simulink model "VCU_Modes"  (R2025b)
settings: Solver=FixedStepDiscrete  StartTime=0.0  StopTime=10.0  FixedStep=0.01  RelTol=1e-3
values from neighbouring files (symbols this model uses):
  c_VCU_BattCurrDrvThd = 100.0    [VCU_Modes.sldd]
  c_VCU_BattCurrDrvTime = 200.0    [VCU_Modes.sldd]
  c_VCU_BattCurrParkThd = 5.0    [VCU_Modes.sldd]
  c_VCU_BattCurrPeakDrvThd = 180.0    [VCU_Modes.sldd]
  c_VCU_BattSocDrvThd = 10.0    [VCU_Modes.sldd]
  c_VCU_BattSocLimpThd = 5.0    [VCU_Modes.sldd]
  c_VCU_BattTempDrvThdMax = 60.0    [VCU_Modes.sldd]
  c_VCU_BattTempParkThd = 45.0    [VCU_Modes.sldd]
  c_VCU_BattTempParkThdFlt = 55.0    [VCU_Modes.sldd]
  c_VCU_DrvThdWait = 100.0    [VCU_Modes.sldd]
  c_VCU_EcuTempDrvThdMax = 95.0    [VCU_Modes.sldd]
  c_VCU_EcuTempParkThd = 70.0    [VCU_Modes.sldd]
  c_VCU_EcuTempParkThdFlt = 85.0    [VCU_Modes.sldd]
  c_VCU_FailSafeThdTime = 200.0    [VCU_Modes.sldd]
  c_VCU_FrontLampExclusive_B = 0.0    [VCU_Modes.sldd]
  c_VCU_HeadLampAmbientThd = 300.0    [VCU_Modes.sldd]
  c_VCU_HeadlampAutoEnable_B = 1.0    [VCU_Modes.sldd]
  c_VCU_HeadlampManualOverride_B = 1.0    [VCU_Modes.sldd]
  c_VCU_LongPressTimeThd = 200.0    [VCU_Modes.sldd]
  c_VCU_MotTempDrvThdMax = 120.0    [VCU_Modes.sldd]
  c_VCU_MotTempParkThd = 80.0    [VCU_Modes.sldd]
  c_VCU_MotTempParkThdFlt = 100.0    [VCU_Modes.sldd]
  c_VCU_ParkExtThdWait = 100.0    [VCU_Modes.sldd]
  c_VCU_ParkThdWait = 100.0    [VCU_Modes.sldd]
  F32_ZERO = 0.0    [VCU_Modes.sldd]
  FALSE = 0.0    [VCU_Modes.sldd]
  TRUE = 1.0    [VCU_Modes.sldd]
  UI8_ZERO = 0.0    [VCU_Modes.sldd]
undefined symbols (not defined in the file or in its folder): POWER_MODE, SIG_STATUS, VCU_MODE
libraries: Sanu_Lib x9, simulink x1
(part 2 of 2)

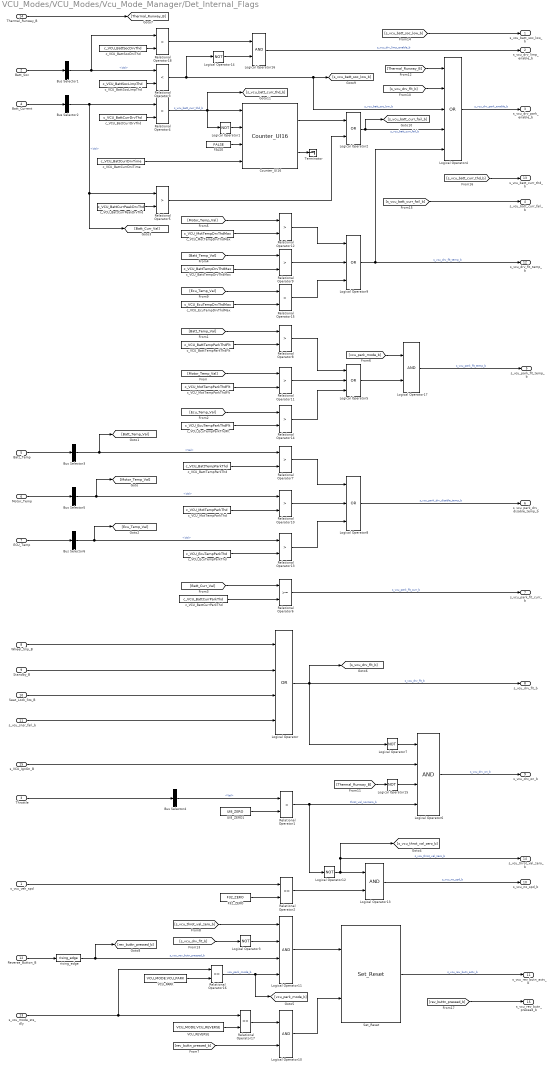
== system VCU_Modes/VCU_Modes/Vcu_Mode_Manager/Det_Internal_Flags ==
  s_vcu_veh_spd : Inport
  Batt_Soc : Inport  Port=2
  Throttle : Inport  Port=3
  Batt_Current : Inport  Port=4
  Batt_Temp : Inport  Port=5
  Motor_Temp : Inport  Port=6
  ECU_Temp : Inport  Port=7
  Wheel_Slip_B : Inport  Port=8
  Standby_B : Inport  Port=9
  Seat_Lock_Sts_B : Inport  Port=10
  s_vcu_snsr_fail_b : Inport  Port=11
  Reverse_Button_B : Inport  Port=12
  s_vcu_mode_sts_dly : Inport  Port=13
  Thermal_Runway_B : Inport  Port=14
  s_VCU_IgnOn_B : Inport  Port=15
  Bus Selector{1..6} (6 alike) : BusSelector  OutputSignals=Val
  Counter_UI16 : Sanu_Lib/Counter_UI16  SystemSampleTime=-1  VariantActivationTime=update diagram  EmptyChoice=off  PassThrough=off  PassThroughVariantControl=(default)  EmptyChoiceVariantControl=(default)  AllowFlexibleInterface=on  Latency=0  AutoFrameSizeCalculation=off
  F32_ZERO : Constant  Value=F32_ZERO  OutDataTypeStr=single  SampleTime=-1
  FALSE : Constant  Value=FALSE  OutDataTypeStr=boolean  SampleTime=-1
  Logical Operator : Logic  Operator=OR  Inputs=4  AllPortsSameDT=off  OutDataTypeStr=boolean
  Logical Operator{1,3,7,12,14..15} (6 alike) : Logic  Operator=NOT  AllPortsSameDT=off  OutDataTypeStr=boolean
  Logical Operator{10,13,16..17} (4 alike) : Logic  AllPortsSameDT=off  OutDataTypeStr=boolean
  Logical Operator11 : Logic  Inputs=4  AllPortsSameDT=off  OutDataTypeStr=boolean
  Logical Operator2 : Logic  Operator=OR  AllPortsSameDT=off  OutDataTypeStr=boolean
  Logical Operator4 : Logic  Operator=OR  Inputs=5  AllPortsSameDT=off  OutDataTypeStr=boolean
  Logical Operator5 : Logic  Operator=OR  Inputs=3  AllPortsSameDT=off  OutDataTypeStr=boolean
  Logical Operator6 : Logic  Inputs=4  AllPortsSameDT=off  OutDataTypeStr=boolean
  Logical Operator8 : Logic  Operator=OR  Inputs=3  AllPortsSameDT=off  OutDataTypeStr=boolean
  Logical Operator9 : Logic  Operator=OR  Inputs=3  AllPortsSameDT=off  OutDataTypeStr=boolean
  Relational Operator{1,4..5,7..15} (12 alike) : RelationalOperator  Operator=>  OutDataTypeStr=boolean  RndMeth=Simplest  InputSameDT=off
  Relational Operator16 : RelationalOperator  Operator===  OutDataTypeStr=boolean  RndMeth=Simplest  InputSameDT=off
  Relational Operator17 : RelationalOperator  Operator===  OutDataTypeStr=boolean  RndMeth=Simplest  InputSameDT=off
  Relational Operator18 : RelationalOperator  Operator=<  OutDataTypeStr=boolean  RndMeth=Simplest  InputSameDT=off
  Relational Operator2 : RelationalOperator  Operator===  OutDataTypeStr=boolean  RndMeth=Simplest  InputSameDT=off
  Relational Operator3 : RelationalOperator  Operator=<  OutDataTypeStr=boolean  RndMeth=Simplest  InputSameDT=off
  Relational Operator6 : RelationalOperator  OutDataTypeStr=boolean  RndMeth=Simplest  InputSameDT=off
  Set_Reset : Sanu_Lib/Set_Reset  SystemSampleTime=-1  VariantActivationTime=update diagram  EmptyChoice=off  PassThrough=off  PassThroughVariantControl=(default)  EmptyChoiceVariantControl=(default)  AllowFlexibleInterface=on  Latency=0  AutoFrameSizeCalculation=off
  Terminator : Terminator
  UI8_ZERO1 : Constant  Value=UI8_ZERO  OutDataTypeStr=uint8  SampleTime=-1
  VCU_PARK : Constant  Value=VCU_MODE.VCU_PARK  OutDataTypeStr=Enum: VCU_MODE  SampleTime=-1
  VCU_REVERSE : Constant  Value=VCU_MODE.VCU_REVERSE  OutDataTypeStr=Enum: VCU_MODE  SampleTime=-1
  c_VCU_BattCurrDrvThd : Constant  Value=c_VCU_BattCurrDrvThd  OutDataTypeStr=single  SampleTime=-1
  c_VCU_BattCurrDrvTime : Constant  Value=c_VCU_BattCurrDrvTime  OutDataTypeStr=uint16  SampleTime=-1
  c_VCU_BattCurrParkThd : Constant  Value=c_VCU_BattCurrParkThd  OutDataTypeStr=single  SampleTime=-1
  c_VCU_BattCurrPeakDrvThd : Constant  Value=c_VCU_BattCurrPeakDrvThd  OutDataTypeStr=single  SampleTime=-1
  c_VCU_BattSocDrvThd : Constant  Value=c_VCU_BattSocDrvThd  OutDataTypeStr=uint8  SampleTime=-1
  c_VCU_BattSocLimpThd : Constant  Value=c_VCU_BattSocLimpThd  OutDataTypeStr=uint8  SampleTime=-1
  c_VCU_BattTempDrvThdMax : Constant  Value=c_VCU_BattTempDrvThdMax  OutDataTypeStr=single  SampleTime=-1
  c_VCU_BattTempParkThd : Constant  Value=c_VCU_BattTempParkThd  OutDataTypeStr=single  SampleTime=-1
  c_VCU_BattTempParkThdFlt : Constant  Value=c_VCU_BattTempParkThdFlt  OutDataTypeStr=single  SampleTime=-1
  c_VCU_EcuTempDrvThdMax : Constant  Value=c_VCU_EcuTempDrvThdMax  OutDataTypeStr=single  SampleTime=-1
  c_VCU_EcuTempParkThd : Constant  Value=c_VCU_EcuTempParkThd  OutDataTypeStr=single  SampleTime=-1
  c_VCU_EcuTempParkThdFlt : Constant  Value=c_VCU_EcuTempParkThdFlt  OutDataTypeStr=single  SampleTime=-1
  c_VCU_MotTempDrvThdMax : Constant  Value=c_VCU_MotTempDrvThdMax  OutDataTypeStr=single  SampleTime=-1
  c_VCU_MotTempParkThd : Constant  Value=c_VCU_MotTempParkThd  OutDataTypeStr=single  SampleTime=-1
  c_VCU_MotTempParkThdFlt : Constant  Value=c_VCU_MotTempParkThdFlt  OutDataTypeStr=single  SampleTime=-1
  rising_edge : Sanu_Lib/rising_edge  SystemSampleTime=-1  VariantActivationTime=update diagram  EmptyChoice=off  PassThrough=off  PassThroughVariantControl=(default)  EmptyChoiceVariantControl=(default)  AllowFlexibleInterface=on  Latency=0  AutoFrameSizeCalculation=off
  s_vcu_batt_soc_low_b : Outport
  s_vcu_drv_limp_enable_b : Outport  Port=2
  s_vcu_drv_park_enable_b : Outport  Port=3
  s_vcu_batt_curr_fail_b : Outport  Port=4
  s_vcu_park_flt_temp_b : Outport  Port=5
  s_vcu_park_drv_disable_temp_b : Outport  Port=6
  s_vcu_park_flt_curr_b : Outport  Port=7
  s_vcu_drv_flt_b : Outport  Port=8
  s_vcu_drv_on_b : Outport  Port=9
  s_vcu_no_spd_b : Outport  Port=10
  s_vcu_rev_butn_actv_b : Outport  Port=11
  s_vcu_drv_flt_temp_b : Outport  Port=12
  s_vcu_batt_curr_thd_b : Outport  Port=13
  s_vcu_throt_val_zero_b : Outport  Port=14
  s_vcu_rev_butn_pressed_b : Outport  Port=15
  wires:
  [s_vcu_batt_soc_low_b] -> s_vcu_batt_soc_low_b/1
  Logical Operator16/1 -> s_vcu_drv_limp_enable_b/1  "s_vcu_drv_limp_enable_b"
  Relational Operator18/1 -> Logical Operator16/1
  Logical Operator14/1 -> Logical Operator16/2
  c_VCU_BattSocDrvThd/1 -> Relational Operator18/2
  [Thermal_Runway_B] -> Logical Operator4/1
  s_VCU_IgnOn_B/1 -> Logical Operator6/2
  Relational Operator6/1 -> s_vcu_park_flt_curr_b/1  "s_vcu_park_flt_curr_b"
  Logical Operator15/1 -> Logical Operator6/3
  [Thermal_Runway_B] -> Logical Operator15/1
  [rev_buttn_pressed_b] -> Logical Operator10/2
  [s_vcu_throt_val_zero_b] -> Logical Operator11/1
  Logical Operator3/1 -> Logical Operator11/2
  [s_vcu_drv_flt_b] -> Logical Operator3/1
  Logical Operator13/1 -> s_vcu_no_spd_b/1  "s_vcu_no_spd_b"
  [Ecu_Temp_Val] -> Relational Operator15/1
  Logical Operator4/1 -> s_vcu_drv_park_enable_b/1  "s_vcu_drv_park_enable_b"
  [Motor_Temp_Val] -> Relational Operator12/1
  Relational Operator9/1 -> Logical Operator9/2
  Logical Operator8/1 -> s_vcu_park_drv_disable_temp_b/1  "s_vcu_park_drv_disable_temp_b"
  Logical Operator/1 -> [s_vcu_drv_flt_b], s_vcu_drv_flt_b/1, Logical Operator7/1  "s_vcu_drv_flt_b"
  FALSE/1 -> Counter_UI16/3
  Relational Operator7/1 -> Logical Operator8/1
  Logical Operator1/1 -> Counter_UI16/2
  [Batt_Temp_Val] -> Relational Operator8/1
  Relational Operator16/1 -> [vcu_park_mode_b], Logical Operator11/4  "vcu_park_mode_b"
  Logical Operator11/1 -> Set_Reset/1
  Logical Operator7/1 -> Logical Operator6/1
  s_vcu_veh_spd/1 -> Relational Operator2/1
  c_VCU_EcuTempParkThdFlt/1 -> Relational Operator14/2
  Bus Selector6/1 -> Relational Operator13/1, [Ecu_Temp_Val]  "<Val>"
  s_vcu_snsr_fail_b/1 -> Logical Operator/4
  c_VCU_BattCurrPeakDrvThd/1 -> Relational Operator5/2
  c_VCU_BattTempParkThd/1 -> Relational Operator7/2
  ECU_Temp/1 -> Bus Selector6/1
  Seat_Lock_Sts_B/1 -> Logical Operator/3
  Logical Operator10/1 -> Set_Reset/2
  Relational Operator13/1 -> Logical Operator8/3
  c_VCU_BattCurrDrvTime/1 -> Counter_UI16/4
  Relational Operator11/1 -> Logical Operator5/2
  Relational Operator12/1 -> Logical Operator9/1
  [Batt_Temp_Val] -> Relational Operator9/1
  Logical Operator9/1 -> s_vcu_drv_flt_temp_b/1, Logical Operator4/5  "s_vcu_drv_flt_temp_b"
  c_VCU_BattCurrParkThd/1 -> Relational Operator6/2
  VCU_REVERSE/1 -> Relational Operator17/2
  Set_Reset/1 -> s_vcu_rev_butn_actv_b/1  "s_vcu_rev_butn_actv_b"
  VCU_PARK/1 -> Relational Operator16/2
  Counter_UI16/1 -> Logical Operator2/1
  [Ecu_Temp_Val] -> Relational Operator14/1
  Bus Selector1/1 -> Relational Operator3/1, Relational Operator18/1  "<Val>"
  Relational Operator2/1 -> Logical Operator13/2
  Relational Operator5/1 -> Logical Operator2/2
  Bus Selector5/1 -> Relational Operator10/1, [Motor_Temp_Val]  "<Val>"
  Batt_Soc/1 -> Bus Selector1/1
  [Motor_Temp_Val] -> Relational Operator11/1
  [s_vcu_drv_flt_b] -> Logical Operator4/2
  c_VCU_BattCurrDrvThd/1 -> Relational Operator4/2
  c_VCU_MotTempDrvThdMax/1 -> Relational Operator12/2
  Bus Selector3/1 -> Relational Operator7/1, [Batt_Temp_Val]  "<Val>"
  Relational Operator1/1 -> Logical Operator6/4, Logical Operator12/1  "throt_val_nonzero_b"
  c_VCU_MotTempParkThdFlt/1 -> Relational Operator11/2
  Batt_Temp/1 -> Bus Selector3/1
  Motor_Temp/1 -> Bus Selector5/1
  Relational Operator10/1 -> Logical Operator8/2
  rising_edge/1 -> Logical Operator11/3, [rev_buttn_pressed_b]  "s_vcu_rev_butn_pressed_b"
  c_VCU_MotTempParkThd/1 -> Relational Operator10/2
  Standby_B/1 -> Logical Operator/2
  Reverse_Button_B/1 -> rising_edge/1
  Wheel_Slip_B/1 -> Logical Operator/1
  Relational Operator17/1 -> Logical Operator10/1
  Throttle/1 -> Bus Selector4/1
  F32_ZERO/1 -> Relational Operator2/2
  [Batt_Curr_Val] -> Relational Operator6/1
  Relational Operator8/1 -> Logical Operator5/1
  c_VCU_BattSocLimpThd/1 -> Relational Operator3/2
  c_VCU_BattTempDrvThdMax/1 -> Relational Operator9/2
  Relational Operator15/1 -> Logical Operator9/3
  Logical Operator2/1 -> Logical Operator4/4, [s_vcu_batt_curr_fail_b]  "s_vcu_batt_curr_fail_b"
  Logical Operator6/1 -> s_vcu_drv_on_b/1  "s_vcu_drv_on_b"
  Counter_UI16/2 -> Terminator/1
  Bus Selector4/1 -> Relational Operator1/1  "<Val>"
  Logical Operator12/1 -> [s_vcu_throt_val_zero_b], s_vcu_throt_val_zero_b/1, Logical Operator13/1  "s_vcu_throt_val_zero_b"
  c_VCU_BattTempParkThdFlt/1 -> Relational Operator8/2
  c_VCU_EcuTempDrvThdMax/1 -> Relational Operator15/2
  Thermal_Runway_B/1 -> [Thermal_Runway_B]
  Relational Operator14/1 -> Logical Operator5/3
  Relational Operator4/1 -> [s_vcu_batt_curr_thd_b], Logical Operator1/1, Counter_UI16/1  "s_vcu_batt_curr_thd_b"
  Bus Selector2/1 -> Relational Operator4/1, Relational Operator5/1, [Batt_Curr_Val]  "<Val>"
  c_VCU_EcuTempParkThd/1 -> Relational Operator13/2
  UI8_ZERO1/1 -> Relational Operator1/2
  Batt_Current/1 -> Bus Selector2/1
  Relational Operator3/1 -> Logical Operator4/3, [s_vcu_batt_soc_low_b], Logical Operator14/1  "s_vcu_batt_soc_low_b"
  s_vcu_mode_sts_dly/1 -> Relational Operator16/1, Relational Operator17/1
  [vcu_park_mode_b] -> Logical Operator17/1
  [s_vcu_batt_curr_fail_b] -> s_vcu_batt_curr_fail_b/1
  [s_vcu_batt_curr_thd_b] -> s_vcu_batt_curr_thd_b/1
  Logical Operator5/1 -> Logical Operator17/2
  Logical Operator17/1 -> s_vcu_park_flt_temp_b/1  "s_vcu_park_flt_temp_b"
  [rev_buttn_pressed_b] -> s_vcu_rev_butn_pressed_b/1

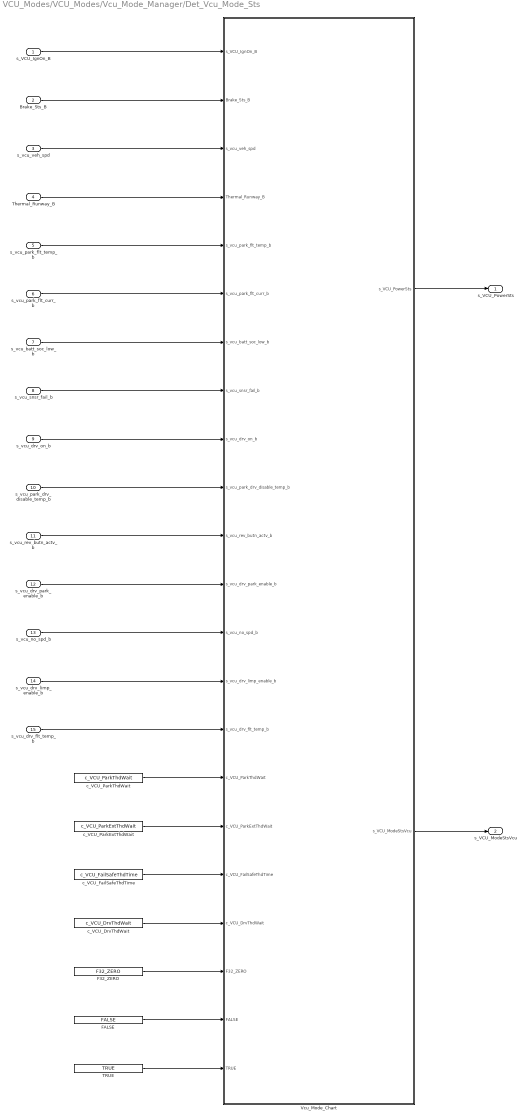
== system VCU_Modes/VCU_Modes/Vcu_Mode_Manager/Det_Vcu_Mode_Sts ==
  s_VCU_IgnOn_B : Inport
  Brake_Sts_B : Inport  Port=2
  s_vcu_veh_spd : Inport  Port=3
  Thermal_Runway_B : Inport  Port=4
  s_vcu_park_flt_temp_b : Inport  Port=5
  s_vcu_park_flt_curr_b : Inport  Port=6
  s_vcu_batt_soc_low_b : Inport  Port=7
  s_vcu_snsr_fail_b : Inport  Port=8
  s_vcu_drv_on_b : Inport  Port=9
  s_vcu_park_drv_disable_temp_b : Inport  Port=10
  s_vcu_rev_butn_actv_b : Inport  Port=11
  s_vcu_drv_park_enable_b : Inport  Port=12
  s_vcu_no_spd_b : Inport  Port=13
  s_vcu_drv_limp_enable_b : Inport  Port=14
  s_vcu_drv_flt_temp_b : Inport  Port=15
  F32_ZERO : Constant  Value=F32_ZERO  OutDataTypeStr=single  SampleTime=-1
  FALSE : Constant  Value=FALSE  OutDataTypeStr=boolean  SampleTime=-1
  TRUE : Constant  Value=TRUE  OutDataTypeStr=boolean  SampleTime=-1
  Vcu_Mode_Chart : Stateflow chart  TreatAsAtomicUnit=on
      settings: PortSchema="{\"entries\":[{\"content\":{\"sides\":[{\"content\":{\"connectorIds\":[\"In1\",\"In2\",\"In3\",\"In4\",\"In5\",\"In6\",\"In7\",\"In8\",\"In9\",\"In10\",\"In11\",\"In12\",\"In13\",\"In14\",\"In15\",\"In16\",\"In18\",\"In17\",\"In19\",\"In20\",\"In21\",\"In22\"]},\"type\":\"ConnectorPlacement.EquallySpacedRectSide\",\"uuid\":\"35025c92-f7ea-4c68-bbf7-eead624e483f\"},{\"content\":{\"connectorIds\":[\"Out1\",\"Out2\"],\"side\":\"RIGHT\"},\"type\":\"ConnectorPlacement.EquallySpacedRectSide\",\"uuid\":\"04b476af-775e-4130-9977-c38802426b78\"},{\"content\":{\"side\":\"TOP\"},\"type\":\"ConnectorPlacement.EquallySpacedRectSide\",\"uuid\":\"5327a217-51d4-4e1d-848e-3c1107d92c88\"}]},\"type\":\"ConnectorPlacement.EquallySpacedConnector\",\"uuid\":\"3867ef37-b688-49f3-9610-30f88bf37bff\"}],\"packageUris\":[\"http://schema.mathworks.com/mf0/Connector/R2020b\"],\"version\":\"1.0\"}"
  c_VCU_DrvThdWait : Constant  Value=c_VCU_DrvThdWait  OutDataTypeStr=uint16  SampleTime=-1
  c_VCU_FailSafeThdTime : Constant  Value=c_VCU_FailSafeThdTime  OutDataTypeStr=uint16  SampleTime=-1
  c_VCU_ParkExtThdWait : Constant  Value=c_VCU_ParkExtThdWait  OutDataTypeStr=uint16  SampleTime=-1
  c_VCU_ParkThdWait : Constant  Value=c_VCU_ParkThdWait  OutDataTypeStr=uint16  SampleTime=-1
  s_VCU_PowerSts : Outport
  s_VCU_ModeStsVcu : Outport  Port=2
  wires:
  s_VCU_IgnOn_B/1 -> Vcu_Mode_Chart/1(s_VCU_IgnOn_B)
  Brake_Sts_B/1 -> Vcu_Mode_Chart/2(Brake_Sts_B)
  Vcu_Mode_Chart/2(" s_VCU_ModeStsVcu") -> s_VCU_ModeStsVcu/1
  Vcu_Mode_Chart/1(s_VCU_PowerSts) -> s_VCU_PowerSts/1
  s_vcu_veh_spd/1 -> Vcu_Mode_Chart/3(s_vcu_veh_spd)
  Thermal_Runway_B/1 -> Vcu_Mode_Chart/4(Thermal_Runway_B)
  s_vcu_park_flt_temp_b/1 -> Vcu_Mode_Chart/5(s_vcu_park_flt_temp_b)
  s_vcu_park_flt_curr_b/1 -> Vcu_Mode_Chart/6(s_vcu_park_flt_curr_b)
  s_vcu_batt_soc_low_b/1 -> Vcu_Mode_Chart/7(s_vcu_batt_soc_low_b)
  s_vcu_snsr_fail_b/1 -> Vcu_Mode_Chart/8(s_vcu_snsr_fail_b)
  s_vcu_drv_on_b/1 -> Vcu_Mode_Chart/9(s_vcu_drv_on_b)
  s_vcu_park_drv_disable_temp_b/1 -> Vcu_Mode_Chart/10(s_vcu_park_drv_disable_temp_b)
  s_vcu_rev_butn_actv_b/1 -> Vcu_Mode_Chart/11(s_vcu_rev_butn_actv_b)
  s_vcu_drv_park_enable_b/1 -> Vcu_Mode_Chart/12(s_vcu_drv_park_enable_b)
  s_vcu_no_spd_b/1 -> Vcu_Mode_Chart/13(s_vcu_no_spd_b)
  s_vcu_drv_limp_enable_b/1 -> Vcu_Mode_Chart/14(s_vcu_drv_limp_enable_b)
  F32_ZERO/1 -> Vcu_Mode_Chart/20(F32_ZERO)
  s_vcu_drv_flt_temp_b/1 -> Vcu_Mode_Chart/15(s_vcu_drv_flt_temp_b)
  FALSE/1 -> Vcu_Mode_Chart/21(FALSE)
  TRUE/1 -> Vcu_Mode_Chart/22(TRUE)
  c_VCU_ParkExtThdWait/1 -> Vcu_Mode_Chart/18(c_VCU_ParkExtThdWait)
  c_VCU_ParkThdWait/1 -> Vcu_Mode_Chart/16(c_VCU_ParkThdWait)
  c_VCU_FailSafeThdTime/1 -> Vcu_Mode_Chart/17(c_VCU_FailSafeThdTime)
  c_VCU_DrvThdWait/1 -> Vcu_Mode_Chart/19(c_VCU_DrvThdWait)

== stateflow chart VCU_Modes/Vcu_Drive_Modes/Drive_Modes ==
  settings: executeAtInitialization=1
  state DRV_OFF
  state DRV_NORMAL
  state DRV_ECO
  state DRV_SPORT
  state DRV_TURBO
  (default) -> DRV_OFF
  DRV_OFF -> DRV_NORMAL : [s_VCU_ModeStsVcu == VCU_MODE.VCU_DRIVE || ...
      | s_VCU_ModeStsVcu == VCU_MODE.VCU_REVERSE]
  DRV_NORMAL -> DRV_OFF [order 1] : [s_VCU_ModeStsVcu == VCU_MODE.VCU_PARK]
  (junction 40) -> DRV_OFF : [s_VCU_ModeStsVcu == VCU_MODE.VCU_PARK]
  DRV_NORMAL -> DRV_ECO [order 2] : [s_VCU_ModeStsVcu == VCU_MODE.VCU_LIMP || ...
      | Mode_Selection == MODE_SELECT.MODE_ECO]
  DRV_ECO -> DRV_NORMAL [order 2] : [Mode_Selection == MODE_SELECT.MODE_NORMAL && ...
      | s_VCU_ModeStsVcu != VCU_MODE.VCU_LIMP]
  DRV_NORMAL -> DRV_SPORT [order 3] : [Mode_Selection == ...
      | MODE_SELECT.MODE_SPORT]
  DRV_NORMAL -> (junction 34) [order 4]
  DRV_ECO -> DRV_SPORT [order 3] : [Mode_Selection == MODE_SELECT.MODE_SPORT && ...
      | s_VCU_ModeStsVcu != VCU_MODE.VCU_LIMP]
  DRV_SPORT -> (junction 34) [order 1]
  (junction 34) -> (junction 47) [order 1]
  (junction 34) -> DRV_TURBO [order 2] : [Mode_Selection == MODE_SELECT.MODE_TURBO]
  (junction 47) -> (junction 51)
  (junction 28) -> DRV_ECO : [Mode_Selection == MODE_SELECT.MODE_ECO || ...
      | s_VCU_ModeStsVcu == VCU_MODE.VCU_LIMP]
  DRV_SPORT -> (junction 28) [order 2]
  DRV_TURBO -> (junction 28) [order 2]
  DRV_ECO -> (junction 40) [order 1]
  (junction 44) -> (junction 40)
  DRV_ECO -> DRV_TURBO [order 4] : [Mode_Selection == MODE_SELECT.MODE_TURBO && ...
      | s_VCU_ModeStsVcu != VCU_MODE.VCU_LIMP]
  DRV_TURBO -> (junction 44) [order 1]
  (junction 53) -> (junction 44)
  (junction 51) -> (junction 53)
  data: s_VCU_ModeStsVcu input Enum: VCU_MODE; Mode_Selection input Enum: MODE_SELECT; s_VCU_DriveMode output Enum: VCU_DRV_MODE

== stateflow chart VCU_Modes/Vcu_Dashboard_Display/Dashboard_Display ==
  settings: executeAtInitialization=1
  (default) -> (junction 3)
  (junction 3) -> (junction 5) [order 1] : [s_VCU_ModeStsVcu == VCU_MODE.VCU_WAKE_UP]
  (junction 5) -> (junction 7) : {
      | s_VCU_ModeDisplay = ...
      | VCU_DISPLAY.DISP_INIT;
      | }
  (junction 3) -> (junction 9) [order 2]
  (junction 9) -> (junction 11) [order 1] : [s_vcu_mode_sts_dly == VCU_MODE.VCU_WAKE_UP && ...
      | s_VCU_ModeStsVcu == VCU_MODE.VCU_PARK]
  (junction 11) -> (junction 13) : {
      | s_VCU_ModeDisplay = ...
      | VCU_DISPLAY.DISP_PARK;
      | }
  (junction 9) -> (junction 15) [order 2]
  (junction 15) -> (junction 17) [order 1] : [s_VCU_ModeStsVcu == VCU_MODE.VCU_PARK && ...
      | s_vcu_drv_park_enable_b == TRUE]
  (junction 15) -> (junction 21) [order 2]
  (junction 17) -> (junction 19) : {
      | s_VCU_ModeDisplay = ...
      | VCU_DISPLAY.DISP_PARK_WARN;
      | }
  (junction 21) -> (junction 23) [order 1] : [s_VCU_ModeStsVcu == VCU_MODE.VCU_PARK && ...
      | s_vcu_mode_sts_dly == VCU_MODE.VCU_DRIVE]
  (junction 21) -> (junction 28) [order 2]
  (junction 23) -> (junction 26) : {
      | s_VCU_ModeDisplay = ...
      | VCU_DISPLAY.DISP_PARK;
      | }
  (junction 28) -> (junction 30) [order 1] : [s_VCU_ModeStsVcu == VCU_MODE.VCU_FAIL_SAFE && ...
      | Thermal_Runway_B == TRUE]
  (junction 28) -> (junction 34) [order 2]
  (junction 30) -> (junction 32) : {
      | s_VCU_ModeDisplay = ...
      | VCU_DISPLAY.DISP_FAIL_THERMAL;
      | }
  (junction 34) -> (junction 36) [order 1] : [s_VCU_ModeStsVcu == VCU_MODE.VCU_FAIL_SAFE && ...
      | s_vcu_batt_soc_low_b == TRUE]
  (junction 34) -> (junction 40) [order 2]
  (junction 36) -> (junction 38) : {
      | s_VCU_ModeDisplay = ...
      | VCU_DISPLAY.DISP_FAIL_SOC;
      | }
  (junction 40) -> (junction 42) [order 1] : [s_VCU_ModeStsVcu == VCU_MODE.VCU_FAIL_SAFE && ...
      | s_vcu_snsr_critical_b == TRUE]
  (junction 40) -> (junction 46) [order 2]
  (junction 42) -> (junction 44) : {
      | s_VCU_ModeDisplay = ...
      | VCU_DISPLAY.DISP_FAIL_CRITICAL;
      | }
  (junction 46) -> (junction 48) [order 1] : [s_VCU_ModeStsVcu == VCU_MODE.VCU_FAIL_SAFE && ...
      | s_vcu_snsr_fail_b == TRUE]
  (junction 46) -> (junction 52) [order 2]
  (junction 48) -> (junction 50) : {
      | s_VCU_ModeDisplay = ...
      | VCU_DISPLAY.DISP_FAIL_SNSR;
      | }
  (junction 52) -> (junction 54) [order 1] : [s_VCU_ModeStsVcu == VCU_MODE.VCU_FAIL_SAFE && ...
      | (s_vcu_drv_flt_temp_b == TRUE || ...
      | s_vcu_park_flt_temp_b == TRUE)]
  (junction 52) -> (junction 58) [order 2]
  (junction 54) -> (junction 56) : {
      | s_VCU_ModeDisplay = ...
      | VCU_DISPLAY.DISP_FAIL_TEMP;
      | }
  (junction 58) -> (junction 60) [order 1] : [s_VCU_ModeStsVcu == VCU_MODE.VCU_FAIL_SAFE && ...
      | (s_vcu_park_flt_curr_b == TRUE || ...
      | s_vcu_batt_curr_fail_b == TRUE)]
  (junction 58) -> (junction 64) [order 2]
  (junction 60) -> (junction 62) : {
      | s_VCU_ModeDisplay = ...
      | VCU_DISPLAY.DISP_FAIL_CURR;
      | }
  (junction 64) -> (junction 66) [order 1] : [s_VCU_ModeStsVcu == VCU_MODE.VCU_PARK && ...
      | throt_val_b]
  (junction 66) -> (junction 68) [order 1] : [s_vcu_park_drv_disable_temp_b == TRUE]
  (junction 64) -> (junction 106) [order 2]
  (junction 66) -> (junction 72) [order 2]
  (junction 68) -> (junction 70) : {
      | s_VCU_ModeDisplay = ...
      | VCU_DISPLAY.DISP_PARK_TEMP;
      | }
  (junction 106) -> (junction 108) [order 1] : [s_VCU_ModeStsVcu == VCU_MODE.VCU_LIMP]
  (junction 72) -> (junction 74) [order 1] : [Wheel_Slip_B == TRUE]
  (junction 106) -> (junction 113) [order 2]
  (junction 108) -> (junction 110) : {
      | s_VCU_ModeDisplay = ...
      | VCU_DISPLAY.DISP_DRV_LIMP;
      | }
  (junction 72) -> (junction 78) [order 2]
  (junction 74) -> (junction 76) : {
      | s_VCU_ModeDisplay = ...
      | VCU_DISPLAY.DISP_PARK_WHL;
      | }
  (junction 78) -> (junction 80) [order 1] : [Standby_B == TRUE]
  (junction 113) -> (junction 115) [order 1] : [s_VCU_ModeStsVcu == VCU_MODE.VCU_REVERSE]
  (junction 78) -> (junction 84) [order 2]
  (junction 80) -> (junction 82) : {
      | s_VCU_ModeDisplay = ...
      | VCU_DISPLAY.DISP_PARK_STDBY;
      | }
  (junction 113) -> (junction 120) [order 2]
  (junction 115) -> (junction 117) : {
      | s_VCU_ModeDisplay = ...
      | VCU_DISPLAY.DISP_DRV_REV;
      | }
  (junction 120) -> (junction 122) [order 1] : [s_VCU_DriveMode == VCU_DRV_MODE.DRV_NORMAL]
  (junction 84) -> (junction 86) [order 1] : [Seat_Lock_Sts_B == TRUE]
  (junction 120) -> (junction 127) [order 2]
  (junction 122) -> (junction 124) : {
      | s_VCU_ModeDisplay = ...
      | VCU_DISPLAY.DISP_DRV_NORM;
      | }
  (junction 84) -> (junction 103) [order 2]
  (junction 86) -> (junction 88) : {
      | s_VCU_ModeDisplay = ...
      | VCU_DISPLAY.DISP_PARK_SEAT;
      | }
  (junction 127) -> (junction 129) [order 1] : [s_VCU_DriveMode == VCU_DRV_MODE.DRV_ECO]
  (junction 127) -> (junction 134) [order 2]
  (junction 129) -> (junction 131) : {
      | s_VCU_ModeDisplay = ...
      | VCU_DISPLAY.DISP_DRV_ECO;
      | }
  (junction 134) -> (junction 136) [order 1] : [s_VCU_DriveMode == VCU_DRV_MODE.DRV_SPORT]
  (junction 134) -> (junction 141) [order 2]
  (junction 136) -> (junction 138) : {
      | s_VCU_ModeDisplay = ...
      | VCU_DISPLAY.DISP_DRV_SPORT;
      | }
  (junction 141) -> (junction 143) [order 1] : [s_VCU_DriveMode == VCU_DRV_MODE.DRV_TURBO]
  (junction 141) -> (junction 148) [order 2]
  (junction 143) -> (junction 145) : {
      | s_VCU_ModeDisplay = ...
      | VCU_DISPLAY.DISP_DRV_TURBO;
      | }
  (junction 145) -> (junction 148)
  (junction 138) -> (junction 145)
  (junction 131) -> (junction 138)
  (junction 124) -> (junction 131)
  (junction 117) -> (junction 124)
  (junction 110) -> (junction 117)
  (junction 103) -> (junction 110)
  (junction 88) -> (junction 103)
  (junction 82) -> (junction 88)
  (junction 76) -> (junction 82)
  (junction 70) -> (junction 76)
  (junction 62) -> (junction 70)
  (junction 56) -> (junction 62)
  (junction 50) -> (junction 56)
  (junction 44) -> (junction 50)
  (junction 38) -> (junction 44)
  (junction 32) -> (junction 38)
  (junction 26) -> (junction 32)
  (junction 19) -> (junction 26)
  (junction 13) -> (junction 19)
  (junction 7) -> (junction 13)
  (junction 148) -> (junction 151)
  data: s_VCU_ModeStsVcu input Enum: VCU_MODE; s_vcu_mode_sts_dly input Enum: VCU_MODE; s_VCU_DriveMode input Enum: VCU_DRV_MODE; s_vcu_drv_park_enable_b input boolean; Thermal_Runway_B input boolean; s_vcu_batt_soc_low_b input boolean; s_vcu_snsr_critical_b input boolean; s_vcu_snsr_fail_b input boolean; s_vcu_drv_flt_temp_b input boolean; s_vcu_park_flt_temp_b input boolean; s_vcu_park_flt_curr_b input boolean; s_vcu_batt_curr_fail_b input boolean; s_vcu_park_drv_disable_temp_b input boolean; Wheel_Slip_B input boolean; Standby_B input boolean; Seat_Lock_Sts_B input boolean; throt_val_b input boolean; s_VCU_ModeDisplay output Enum: VCU_DISPLAY; TRUE input boolean

== stateflow chart VCU_Modes/Vcu_Mode_Manager/Det_Vcu_Mode_Sts/Vcu_Mode_Chart ==
  settings: executeAtInitialization=1
  state POWER_OFF
  state POWER_ON
    state VCU_PARK
      en: vcu_cnt = 0;
      VCU_PARK -> (junction 37) [order 1]
      (junction 37) -> (junction 41) [order 1] : [s_vcu_veh_spd == F32_ZERO && ...
          | (s_vcu_batt_soc_low_b == TRUE || ...
          | Thermal_Runway_B == TRUE || ...
          | s_vcu_snsr_fail_b == TRUE || ...
          | s_vcu_drv_flt_temp_b == TRUE)]
      (junction 37) -> (junction 72) [order 2] : {
          | vcu_cnt = 0;
          | }
      (junction 41) -> (junction 43) : {
          | vcu_cnt++;
          | }
      (junction 43) -> (junction 72)
      (junction 72) -> (junction 74)
    state VCU_WAKE_UP
      en: vcu_cnt = 0;
      du: vcu_cnt++;
    state VCU_REVERSE
    state VCU_FAIL_SAFE
      en: vcu_cnt = 0;
      du: vcu_cnt++;
    state VCU_LIMP
      en: vcu_cnt = 0;
      VCU_LIMP -> (junction 92) [order 1]
      (junction 92) -> (junction 96) [order 1] : [Brake_Sts_B == TRUE && ...
          | s_vcu_no_spd_b == TRUE]
      (junction 92) -> (junction 90) [order 2] : {vcu_cnt = 0;}
      (junction 96) -> (junction 97) : {vcu_cnt++;}
      (junction 97) -> (junction 90)
      (junction 90) -> (junction 99)
    state VCU_DRIVE
      en: vcu_cnt = 0;
      VCU_DRIVE -> (junction 20) [order 1]
      (junction 20) -> (junction 22) [order 1] : [Brake_Sts_B == TRUE && ...
          | s_vcu_no_spd_b == TRUE]
      (junction 20) -> (junction 26) [order 2] : {vcu_cnt = 0;}
      (junction 22) -> (junction 24) : {vcu_cnt++;}
      (junction 24) -> (junction 26)
      (junction 26) -> (junction 29)
    (default) -> VCU_WAKE_UP
    VCU_WAKE_UP -> VCU_PARK : [vcu_cnt >= c_VCU_ParkThdWait]
    VCU_PARK -> VCU_REVERSE [order 4] : [s_vcu_rev_butn_actv_b == TRUE]
    VCU_REVERSE -> VCU_PARK [order 1] : [s_vcu_drv_park_enable_b == TRUE || ...
        | s_VCU_IgnOn_B == FALSE]
    VCU_REVERSE -> VCU_PARK [order 2] : [s_vcu_rev_butn_actv_b == TRUE && ...
        | s_vcu_no_spd_b == TRUE]
    VCU_PARK -> VCU_FAIL_SAFE [order 1] : [vcu_cnt >= c_VCU_ParkExtThdWait || ...
        | s_vcu_park_flt_temp_b == TRUE || ...
        | s_vcu_park_flt_curr_b == TRUE]
    VCU_FAIL_SAFE -> VCU_PARK [order 1] : [s_vcu_batt_soc_low_b == FALSE && ...
        | Thermal_Runway_B == FALSE && ...
        | s_vcu_snsr_fail_b == FALSE]
    VCU_PARK -> VCU_DRIVE [order 2] : [s_vcu_drv_on_b == TRUE && ...
        | s_vcu_park_drv_disable_temp_b == FALSE]
    (junction 103) -> VCU_PARK : [s_VCU_IgnOn_B == FALSE || ...
        | vcu_cnt >= c_VCU_DrvThdWait || ...
        | s_vcu_drv_park_enable_b == TRUE]
    VCU_LIMP -> (junction 103) [order 1]
    VCU_DRIVE -> (junction 103) [order 1]
    VCU_DRIVE -> VCU_LIMP [order 2] : [s_vcu_drv_limp_enable_b == TRUE]
  (default) -> POWER_OFF
  POWER_OFF -> POWER_ON : [s_VCU_IgnOn_B == TRUE]
  VCU_PARK -> POWER_OFF [order 3] : [s_VCU_IgnOn_B == FALSE && ...
      | s_vcu_veh_spd == F32_ZERO]
  VCU_FAIL_SAFE -> POWER_OFF [order 2] : [vcu_cnt >= c_VCU_FailSafeThdTime]
  data: s_VCU_PowerSts output Enum: POWER_MODE; s_VCU_ModeStsVcu output Enum: VCU_MODE; s_VCU_IgnOn_B input boolean; Brake_Sts_B input boolean; s_vcu_veh_spd input single; Thermal_Runway_B input boolean; s_vcu_park_flt_temp_b input boolean; s_vcu_park_flt_curr_b input boolean; s_vcu_batt_soc_low_b input boolean; s_vcu_snsr_fail_b input boolean; s_vcu_drv_on_b input boolean; s_vcu_park_drv_disable_temp_b input boolean; s_vcu_rev_butn_actv_b input boolean; s_vcu_drv_park_enable_b input boolean; s_vcu_no_spd_b input boolean; s_vcu_drv_limp_enable_b input boolean; s_vcu_drv_flt_temp_b input boolean; c_VCU_ParkThdWait input uint16; c_VCU_FailSafeThdTime input uint16; c_VCU_ParkExtThdWait input uint16; c_VCU_DrvThdWait input uint16; F32_ZERO input single; vcu_cnt local uint16; FALSE input boolean; TRUE input boolean
  data vcu_cnt settings: description=vcu_cnt
